simulink library "carnot"  (R2018b)
settings: Solver=VariableStepAuto  StartTime=0.0  StopTime=10.0  RelTol=1e-3
undefined symbols (not defined in the file or in its folder): A, A_earth, acol, Acol, ActPower1, ActPower2, ActPower3, Ad, Ad0, Ar, Au, Au0, Azimuth_Angle, B, Bd, Bd0, Br, Bu, Bu0, C, c1, c2, c3, c33, c4, c5, c6, CarnotCallbacks_Density, CarnotCallbacks_Enthalpy, CarnotCallbacks_Enthalpy2Temperature, CarnotCallbacks_Entropy, CarnotCallbacks_Evaporation_Enthalpy, CarnotCallbacks_GlobalMessageLevel, CarnotCallbacks_Grashof, CarnotCallbacks_Heat_Capacity, CarnotCallbacks_Kinematic_Viscosity, CarnotCallbacks_PMV_PPD, CarnotCallbacks_Prandtl, CarnotCallbacks_Saturation_Property, CarnotCallbacks_Saturation_Temperature, CarnotCallbacks_Saturation_Value_Water, CarnotCallbacks_Specific_Volume, CarnotCallbacks_Thermal_Conductivity, CarnotCallbacks_Vapour_Content, CarnotCallbacks_Vapour_Pressure, Cd, Cdl, Cr, Cu, Davies, Dd, DE_TRY2010_04_averageYear, delta_grd, density, DiameterLastPiece, dl, DPConstant, DPLinear, DPQuadratic, Dr ... (+59)
libraries: $bdroot x429, simulink x36, simulink_extras x12
(part 15 of 22)

== system carnot/Load/Hot_Water_Tapping/mdot_annual_profile ==
  note: Don't change any names
      | in this subsystem!
  Gain : Gain  Gain=1/10000  SaturateOnIntegerOverflow=on  OutDataTypeStr=Inherit: Same as input  ParamDataTypeStr=Inherit: Same as input
  Multiport Switch : MultiPortSwitch  Inputs=2  SaturateOnIntegerOverflow=on  InputSameDT=on
  Product : Product  Inputs=3  SaturateOnIntegerOverflow=on  InputSameDT=on  OutDataTypeStr=Inherit: Same as first input
  RS Month : simulink/Sources/Repeating Sequence  rep_seq_t=[0 2678399 2678399+1 5097599 5097599+1 7775999 7775999+1 10367999 10367999+1 13046399 13046399+1 15638399 15638399+1 18316799 18316799+1 20995199 20995199+1 23587199 23587199+1 26265599 26265599+1 28857599 28857599+1 31536000]  rep_seq_y=[99 99 97 97 100 100 100 100 103 103 105 105 109 109 112 112 108 108 105 105 101 101 100 100]
  RS Sunday : simulink/Sources/Repeating Sequence  rep_seq_t="100*[0 18 18+1 36 36+1 54 54+1 72 72+1 90 90+1 108 108+1 126 126+1 144 144+1 162 162+1 180 180+1 198 198+1 216 216+1 234 234+1 252 252+1 270 270+1 288 288+1 306 306+1 324 324+1 342 342+1 360 360+1 378 378+1 396 396+1 414 414+1 432 432+1 450 450+1 468 468+1 486 486+1 504 504+1 522 522+1 540 540+1 558 558+1 576 576+1 594 594+1 612 612+1 630 630+1 648 648+1 666 666+1 684 684+1 702 702+1 720 720+1 738 738+1 756 756+1 774 774+1 792 792+1 810 810+1 828 828+1 846 846+1  864]"  rep_seq_y=[0 0 0 0 0.5 0.5 0.5 0.5 0.5 0.5 0.5 0.5 1 1 1 1 1 1 1 1 1 1 1 1 1 1 2 2 2 2 3 3 2 2 2 2 2 2 2 2 3 3 2 2 2 2 2 2 3 3 3 3 3 3 3 3 3 3 2 2 2 2 1 1 1 1 2 2 2 2 3 3 3 3 3 3 3 3 2 2 2 2 2 2 2 2 2 2 1 1 1 1 1 1 1 1]
  RS Weekday : simulink/Sources/Repeating Sequence  rep_seq_t="100*[0 18 18+1 36 36+1 54 54+1 72 72+1 90 90+1 108 108+1 126 126+1 144 144+1 162 162+1 180 180+1 198 198+1 216 216+1 234 234+1 252 252+1 270 270+1 288 288+1 306 306+1 324 324+1 342 342+1 360 360+1 378 378+1 396 396+1 414 414+1 432 432+1 450 450+1 468 468+1 486 486+1 504 504+1 522 522+1 540 540+1 558 558+1 576 576+1 594 594+1 612 612+1 630 630+1 648 648+1 666 666+1 684 684+1 702 702+1 720 720+1 738 738+1 756 756+1 774 774+1 792 792+1 810 810+1 828 828+1 846 846+1  864]"  rep_seq_y=[0.5 0.5 0.5 0.5 0.5 0.5 0.5 0.5 0.5 0.5 0.5 0.5 1 1 1 1 1 1 1 1 2 2 2 2 3 3 3 3 5 5 5 5 5 5 5 5 4 4 4 4 3 3 2 2 2 2 2 2 3 3 3 3 4 4 4 4 3 3 2 2 2 2 1 1 1 1 2 2 2 2 3 3 3 3 3 3 3 3 2 2 2 2 2 2 2 2 2 2 1 1 1 1 1 1 1 1]
  Repeating Sequence Day of the Week : simulink/Sources/Repeating Sequence  rep_seq_t=[0 5*24*3600 5*24*3600+1 7*24*3600]  rep_seq_y=[1 1 2 2]
  mdot0 : Constant  Value=0.1
  mdot : Outport
  wires:
  RS Month/1 -> Product/2
  RS Weekday/1 -> Multiport Switch/2
  Gain/1 -> mdot/1
  Product/1 -> Gain/1
  mdot0/1 -> Product/1
  Multiport Switch/1 -> Product/3
  RS Sunday/1 -> Multiport Switch/3
  Repeating Sequence Day of the Week/1 -> Multiport Switch/1

== system carnot/Load/Hot_Water_Tapping/mdot_rep_seq ==
  Add : Sum  Inputs=1
  Pulse Generator : DiscretePulseGenerator  PulseType=Time based  Amplitude=rep_seq_y  Period=period  PulseWidth=rep_seq_d*100/period  PhaseDelay=rep_seq_t
  Out1 : Outport
  wires:
  Pulse Generator/1 -> Add/1
  Add/1 -> Out1/1

== system carnot/Load/Houses/House_simple ==
  WDB : Inport
  THB : Inport  Port=2
  RDB : Inport  Port=3
  Ahabit : Constant  Value=Ahabit
  AirComposition : Subsystem
  Bus Creator : BusCreator  Inputs=8
  Bus Selector1 : BusSelector  OutputSignals=Sunshade,OpenWindow,Qdot_internal
  Bus Selector2 : BusSelector  OutputSignals=CalculateAirComposition
  Constant1 : Constant  Value=20
  HeatTransfer2Ground_ISO13370 : $bdroot/Basic/Heat_Transfer/HeatTransfer2Ground_ISO13370  slabwidth=slabwidth  slablength=slablength  gammat=gammat  Tmeaninside=Tmeaninside  deltathetai=deltathetai  Tmeanoutside=Tmeanoutside  deltathetae=deltathetae  tshift=tshift  dwall=dwall  cond_ground=cond_ground  cp_ground=cp_ground  rho_ground=rho_ground  utot=utot
  House_OneNodeModel : $bdroot/Basic/Thermal_Models/House_OneNodeModel  A=Ahabit  UAout=UAwall  UAin=0  capa=capa  tini=tini  dtroom=dtroom  AziWin=AziWin  Awin=Awindow  Uwin=Uwindow  Gwin=Gwindow
  Radiator : $bdroot/Source/Heat_Exchanger/Radiator  pnom=pnom  dtnom=dtnom  expo=expo  mcap=mcap  tini=tini  lin=lin  qua=qua
  Ventilation : $bdroot/Source/Ventilation/Ventilation  Ahabit=Ahabit  Hroom=Hroom  vent=Ventilationrate  rec=Heatrecovery  ppmCO2=400  ppmVOC=0  alpha=alpha  H=H  W=W  Nwin=Nwin
  Hdat : Outport
  THBout : Outport  Port=2
  wires:
  Ventilation/2 -> AirComposition/1(THBvent)
  AirComposition/1(AirComp) -> Bus Creator/8  "AirComposition"
  Bus Selector2/1 -> AirComposition/Enable  "<CalculateAirComposition>"
  Ahabit/1 -> Bus Creator/7  "Ahabit"
  THB/1 -> Radiator/2, Bus Creator/5  "THB_in"
  Radiator/2 -> THBout/1, Bus Creator/6  "THB_out"
  House_OneNodeModel/1 -> Ventilation/2, Radiator/1, Bus Creator/1  "Troom"
  House_OneNodeModel/2 -> Bus Creator/2  "Qdot"
  Bus Creator/1 -> Hdat/1
  HeatTransfer2Ground_ISO13370/1 -> House_OneNodeModel/5
  Constant1/1 -> House_OneNodeModel/1
  Bus Selector1/3 -> House_OneNodeModel/6  "<Qdot_internal>"
  Radiator/1 -> House_OneNodeModel/7  "Qdot"
  Ventilation/1 -> House_OneNodeModel/4
  WDB/1 -> Ventilation/1, House_OneNodeModel/2, Bus Creator/4  "WDB"
  RDB/1 -> Bus Selector1/1, Bus Selector2/1, AirComposition/2(RDB), Bus Creator/3  "RDB"
  Bus Selector1/1 -> House_OneNodeModel/3  "<Sunshade>"
  Bus Selector1/2 -> Ventilation/3  "<OpenWindow>"

== system carnot/Load/Houses/Resident_Data ==
  Qdot_internal : Inport
  Sunshade : Inport  Port=2
  OpenWindow : Inport  Port=3
  Massflow_CO2 : Inport  Port=4
  Massflow_H2O : Inport  Port=5
  Massflow_VOC : Inport  Port=6
  Bus Creator : BusCreator  Inputs=7
  CalculateAirComposition : Constant  Value=CalcAirComp  mask{CalcAirComp=on}
      mask prompts: CalcAirComp "Calculate the composition of room air (H2O, CO2, VOC)"
  RDB : Outport
  wires:
  CalculateAirComposition/1 -> Bus Creator/4  "CalculateAirComposition"
  Massflow_VOC/1 -> Bus Creator/7  "Massflow_VOC"
  Massflow_H2O/1 -> Bus Creator/6  "Massflow_H2O"
  Massflow_CO2/1 -> Bus Creator/5  "Massflow_CO2"
  Qdot_internal/1 -> Bus Creator/1  "Qdot_internal"
  OpenWindow/1 -> Bus Creator/3  "OpenWindow"
  Bus Creator/1 -> RDB/1
  Sunshade/1 -> Bus Creator/2  "Sunshade"

== system carnot/Load/Houses/Resident_Task44 ==
  WDB : Inport
  Troom : Inport  Port=2
  Bus Creator : BusCreator  Inputs=7
  Bus Selector : BusSelector  OutputSignals=Temperature_Ambient
  CalculateAirComposition : Constant  Value=CalcAirComp  mask{CalcAirComp=off}
      mask prompts: CalcAirComp "Calculate the composition of room air (H2O, CO2, VOC)"
  Electric_Gains_Profile : $bdroot/Load/General/Repeating_Profile  period=period  rep_seq_t=rep_seq_te  rep_seq_d=rep_seq_de  rep_seq_y=rep_seq_ye
  Massflow_CO2 : Constant  Value=mdotCO2
  Massflow_H2O : Constant  Value=mdotH2O
  Massflow_VOC : Constant  Value=mdotVOC
  Occupation_Profile : $bdroot/Load/General/Repeating_Profile  period=period  rep_seq_t=rep_seq_to  rep_seq_d=rep_seq_do  rep_seq_y=rep_seq_yo
  Shading_Control : $bdroot/Control/Shading_Control  TroomShadeOn=TroomShadeOn  TroomShadeOff=TroomShadeOff  SolarShadeOn=SolarShadeOn  SolarShadeOff=SolarShadeOff  max_shade=max_shade
  Window_Control : $bdroot/Control/Window_Control  Topen=Topen  Tclose=Tclose  TrAboveTa=TrAboveTa  TaTooCold=TaTooCold  timeFIR=timeFIR  TaIni=TaIni  starttime=starttime  stoptime=stoptime
  add : Sum  Inputs=2
  RDB : Outport
  wires:
  CalculateAirComposition/1 -> Bus Creator/4  "CalculateAirComposition"
  Massflow_VOC/1 -> Bus Creator/7  "Massflow_VOC"
  Massflow_H2O/1 -> Bus Creator/6  "Massflow_H2O"
  Massflow_CO2/1 -> Bus Creator/5  "Massflow_CO2"
  Occupation_Profile/1 -> add/1
  Electric_Gains_Profile/1 -> add/2
  add/1 -> Bus Creator/1  "Qdot_internal"
  Window_Control/1 -> Bus Creator/3  "OpenWindow"
  Bus Creator/1 -> RDB/1
  Shading_Control/1 -> Bus Creator/2  "Sunshade"
  Bus Selector/1 -> Window_Control/1  "<Temperature_Ambient>"
  Troom/1 -> Window_Control/2, Shading_Control/2
  WDB/1 -> Bus Selector/1, Shading_Control/1

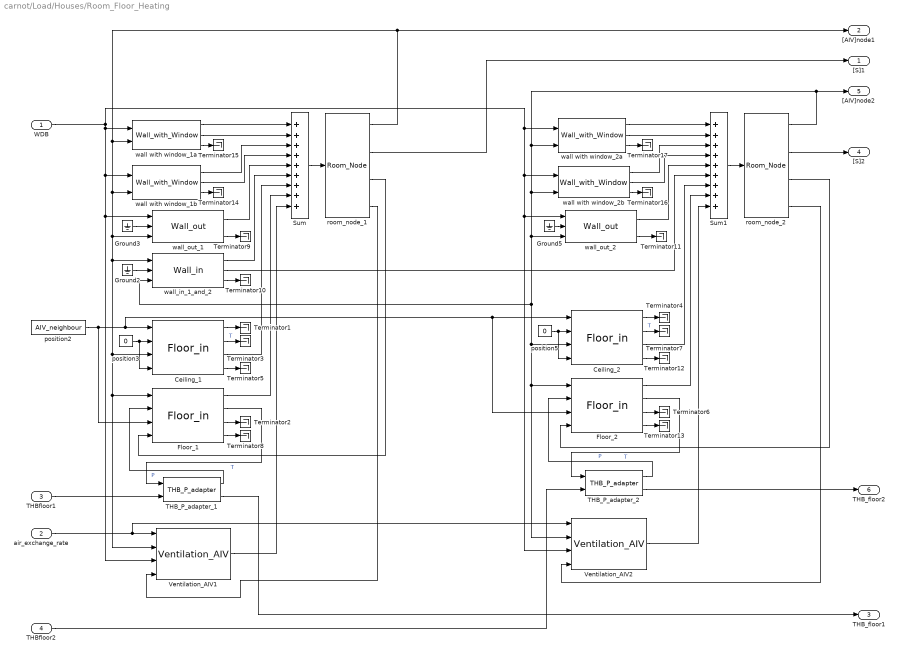
== system carnot/Load/Houses/Room_Floor_Heating ==
  WDB : Inport
  air_exchange_rate : Inport  Port=2
  THBfloor1 : Inport  Port=3
  THBfloor2 : Inport  Port=4
  Ceiling_1 : $bdroot/Basic/Thermal_Models/Floor_in  wallsize=[5 5]  t0=20  d=[0.015 0.38 0.02]  cond=[1.4 0.79 0.7]  cwall=[0.28 0.28 0.28]*3600  rho=[2000 1800 1400]  misc=[0.9 0.9]  dactive=-1  tau=1000*3600
  Ceiling_2 : $bdroot/Basic/Thermal_Models/Floor_in  wallsize=[5 5]  t0=20  d=[0.015 0.38 0.02]  cond=[1.4 0.79 0.7]  cwall=[0.28 0.28 0.28]*3600  rho=[2000 1800 1400]  misc=[0.9 0.9]  dactive=-1  tau=1000*3600
  Floor_1 : $bdroot/Basic/Thermal_Models/Floor_in  wallsize=[5 5]  t0=20  d=[0.015 0.38 0.02]  cond=[1.4 0.79 0.7]  cwall=[0.28 0.28 0.28]*3600  rho=[2000 1800 1400]  misc=[0.9 0.9]  dactive=0.02  tau=1000*3600
  Floor_2 : $bdroot/Basic/Thermal_Models/Floor_in  wallsize=[5 5]  t0=20  d=[0.015 0.38 0.02]  cond=[1.4 0.79 0.7]  cwall=[0.28 0.28 0.28]*3600  rho=[2000 1800 1400]  misc=[0.9 0.9]  dactive=0.02  tau=1000*3600
  Ground2 : Ground
  Ground3 : Ground
  Ground5 : Ground
  Sum : Sum  Inputs=9  SaturateOnIntegerOverflow=on  InputSameDT=on  OutDataTypeStr=Inherit: Same as first input
  Sum1 : Sum  Inputs=9  SaturateOnIntegerOverflow=on  InputSameDT=on  OutDataTypeStr=Inherit: Same as first input
  THB_P_adapter_1 : $bdroot/Source/Heat_Exchanger/THB_P_adapter  mass=1  ua=800*5*5/0.2*0.022*3.1415  t0=20
  THB_P_adapter_2 : $bdroot/Source/Heat_Exchanger/THB_P_adapter  mass=1  ua=800*5*5/0.2*0.022*3.1415  t0=20
  Terminator{1..17} (17 alike) : Terminator
  Ventilation_AIV1 : $bdroot/Source/Ventilation/Ventilation_AIV  co2=400
  Ventilation_AIV2 : $bdroot/Source/Ventilation/Ventilation_AIV  co2=400
  position2 : Constant  Value=AIV_neighbour
  position3 : Constant  Value=0
  position5 : Constant  Value=0
  room_node_1 : $bdroot/Basic/Thermal_Models/Room_Node  zoneairvolume=5*5*2.5  zoneheight=2.5  zonestartTEMP=20  zonestartWATER=55  timeconst=100  heatperfect=natural  lookuptime=[0 24]*3600  lookupvalue=[20 20]  AirPressure=101300  calc_p=off
  room_node_2 : $bdroot/Basic/Thermal_Models/Room_Node  zoneairvolume=5*5*2.5  zoneheight=2.5  zonestartTEMP=20  zonestartWATER=55  timeconst=100  heatperfect=natural  lookuptime=[0 24]*3600  lookupvalue=[20 20]  AirPressure=101300  calc_p=off
  wall with window_1a : $bdroot/Basic/Thermal_Models/Wall_with_Window  wallsize=[2.5 5]  windowsize=[1 2]  frame=0.1  pos=90  t0=20  tau=1000*3600  g=0.7
  wall with window_1b : $bdroot/Basic/Thermal_Models/Wall_with_Window  wallsize=[2.5 5]  windowsize=[1 2]  frame=0.1  pos=0  t0=20  tau=1000*3600  g=0.7
  wall with window_2a : $bdroot/Basic/Thermal_Models/Wall_with_Window  wallsize=[2.5 5]  windowsize=[1 2]  frame=0.1  pos=-90  t0=20  tau=1000*3600  g=0.7
  wall with window_2b : $bdroot/Basic/Thermal_Models/Wall_with_Window  wallsize=[2.5 5]  windowsize=[1 2]  frame=0.1  pos=0  t0=20  tau=1000*3600  g=0.7
  wall_in_1_and_2 : $bdroot/Basic/Thermal_Models/Wall_in  wallsize=[2.5 5]  d=[0.015 0.38 0.02]  cond=[1.4 0.79 0.7]  cwall=[0.28 0.28 0.28]*3600  rho=[2000 1800 1400]  emission_in=.96  dactive=-1  t0=20  tau=1000*3600
  wall_out_1 : $bdroot/Basic/Thermal_Models/Wall_out  wallsize=[2.5 5]  pos=180  t0=20  d=[0.1 0.38]  cond=[0.04 0.79]  cwall=[0.28 0.28]*3600  rho=[900 1800]  reflectground=0.2  abs_emiss=[0.65 0.97 0.96]  tau=1000*3600  dactive=-1
  wall_out_2 : $bdroot/Basic/Thermal_Models/Wall_out  wallsize=[2.5 5]  pos=180  t0=20  d=[0.1 0.38]  cond=[0.04 0.79]  cwall=[0.28 0.28]*3600  rho=[900 1800]  reflectground=0.2  abs_emiss=[0.65 0.97 0.96]  tau=1000*3600  dactive=-1
  "[S]1" : Outport
  "[AIV]node1" : Outport  Port=2
  THB_floor1 : Outport  Port=3
  "[S]2" : Outport  Port=4
  "[AIV]node2" : Outport  Port=5
  THB_floor2 : Outport  Port=6
  wires:
  Sum1/1 -> room_node_2/1
  Sum/1 -> room_node_1/1
  room_node_2/1 -> "[AIV]node2"/1, wall with window_2a/2, wall_in_1_and_2/3, Ceiling_2/3, Ventilation_AIV2/2, Floor_2/1, wall_out_2/3, wall with window_2b/2
  room_node_1/1 -> "[AIV]node1"/1, wall_out_1/3, Ventilation_AIV1/2, Floor_1/1, Ceiling_1/3, wall_in_1_and_2/1, wall with window_1b/2, wall with window_1a/2
  air_exchange_rate/1 -> Ventilation_AIV1/1, Ventilation_AIV2/1
  wall_in_1_and_2/2 -> Sum1/6
  Ground5/1 -> wall_out_2/2
  room_node_2/3 -> Floor_2/4
  room_node_2/4 -> Ventilation_AIV2/4
  THB_P_adapter_2/2 -> THB_floor2/1
  THB_P_adapter_2/1 -> Floor_2/2  "P"
  Floor_2/2 -> THB_P_adapter_2/1  "T"
  THBfloor2/1 -> THB_P_adapter_2/2
  Ventilation_AIV2/1 -> Sum1/9
  Ceiling_2/3 -> Sum1/7
  Floor_2/1 -> Sum1/8
  position5/1 -> Ceiling_2/2, Ceiling_2/4
  Floor_2/3 -> Terminator6/1
  Ceiling_2/2 -> Terminator7/1  "T"
  Ceiling_2/1 -> Terminator4/1
  room_node_2/2 -> "[S]2"/1
  wall with window_2b/2 -> Sum1/4
  wall_out_2/1 -> Sum1/5
  wall with window_2b/1 -> Sum1/3
  wall with window_2a/2 -> Sum1/2
  wall with window_2a/1 -> Sum1/1
  position2/1 -> Ceiling_2/1, Floor_2/3, Ceiling_1/1, Floor_1/3
  Ground3/1 -> wall_out_1/2
  Ground2/1 -> wall_in_1_and_2/2
  room_node_1/3 -> Floor_1/4
  room_node_1/4 -> Ventilation_AIV1/4
  THB_P_adapter_1/2 -> THB_floor1/1
  THB_P_adapter_1/1 -> Floor_1/2  "P"
  Floor_1/2 -> THB_P_adapter_1/1  "T"
  THBfloor1/1 -> THB_P_adapter_1/2
  Ventilation_AIV1/1 -> Sum/9
  Ceiling_1/3 -> Sum/7
  Floor_1/1 -> Sum/8
  position3/1 -> Ceiling_1/4, Ceiling_1/2
  Floor_1/3 -> Terminator2/1
  Ceiling_1/2 -> Terminator3/1  "T"
  Ceiling_1/1 -> Terminator1/1
  room_node_1/2 -> "[S]1"/1
  wall with window_1b/2 -> Sum/4
  wall_out_1/1 -> Sum/5
  wall with window_1b/1 -> Sum/3
  wall with window_1a/2 -> Sum/2
  wall with window_1a/1 -> Sum/1
  WDB/1 -> wall with window_1a/1, Ventilation_AIV1/3, wall_out_1/1, wall with window_1b/1, Ventilation_AIV2/3, wall_out_2/1, wall with window_2b/1, wall with window_2a/1
  wall_in_1_and_2/1 -> Sum/6
  Ceiling_1/4 -> Terminator5/1
  Floor_1/4 -> Terminator8/1
  wall_out_1/2 -> Terminator9/1
  wall_in_1_and_2/3 -> Terminator10/1
  wall_out_2/2 -> Terminator11/1
  Ceiling_2/4 -> Terminator12/1
  Floor_2/4 -> Terminator13/1
  wall with window_1b/3 -> Terminator14/1
  wall with window_1a/3 -> Terminator15/1
  wall with window_2b/3 -> Terminator16/1
  wall with window_2a/3 -> Terminator17/1

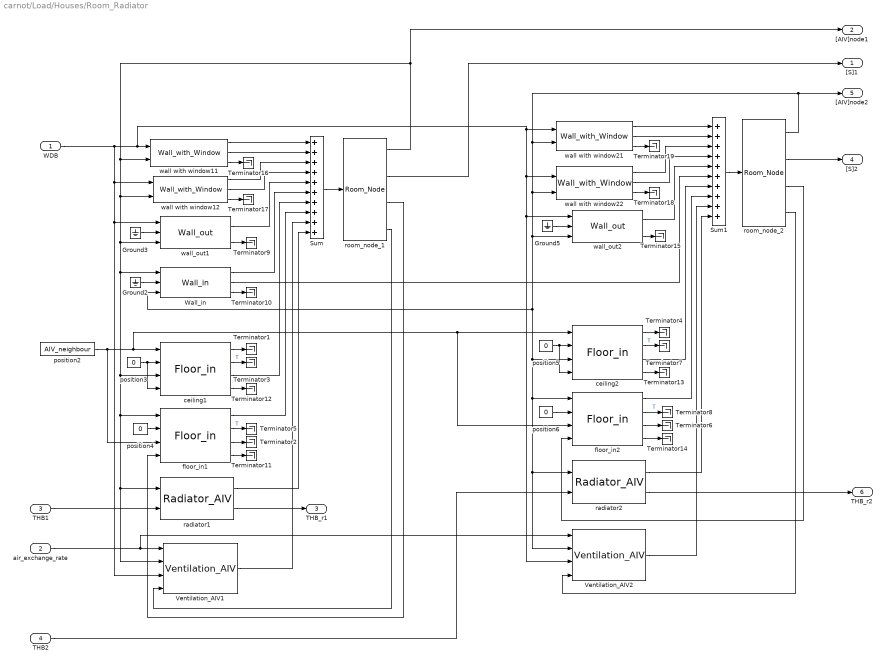
== system carnot/Load/Houses/Room_Radiator ==
  WDB : Inport
  air_exchange_rate : Inport  Port=2
  THB1 : Inport  Port=3
  THB2 : Inport  Port=4
  Ground2 : Ground
  Ground3 : Ground
  Ground5 : Ground
  Sum : Sum  Inputs=10  SaturateOnIntegerOverflow=on  InputSameDT=on  OutDataTypeStr=Inherit: Same as first input
  Sum1 : Sum  Inputs=10  SaturateOnIntegerOverflow=on  InputSameDT=on  OutDataTypeStr=Inherit: Same as first input
  Terminator{1..19} (19 alike) : Terminator
  Ventilation_AIV1 : $bdroot/Source/Ventilation/Ventilation_AIV  co2=400
  Ventilation_AIV2 : $bdroot/Source/Ventilation/Ventilation_AIV  co2=400
  Wall_in : $bdroot/Basic/Thermal_Models/Wall_in  wallsize=[2.5 5]  d=[0.015 0.38 0.02]  cond=[1.4 0.79 0.7]  cwall=[0.28 0.28 0.28]*3600  rho=[2000 1800 1400]  emission_in=0.96  dactive=-1  t0=20  tau=1000*3600
  ceiling1 : $bdroot/Basic/Thermal_Models/Floor_in  wallsize=[5 5]  t0=20  d=[0.015 0.38 0.02]  cond=[1.4 0.79 0.7]  cwall=[0.28 0.28 0.28]*3600  rho=[2000 1800 1400]  misc=[0.9 0.9]  dactive=-1  tau=1000*3600
  ceiling2 : $bdroot/Basic/Thermal_Models/Floor_in  wallsize=[5 5]  t0=20  d=[0.015 0.38 0.02]  cond=[1.4 0.79 0.7]  cwall=[0.28 0.28 0.28]*3600  rho=[2000 1800 1400]  misc=[0.9 0.9]  dactive=-1  tau=1000*3600
  floor_in1 : $bdroot/Basic/Thermal_Models/Floor_in  wallsize=[5 5]  t0=20  d=[0.015 0.38 0.02]  cond=[1.4 0.79 0.7]  cwall=[0.28 0.28 0.28]*3600  rho=[2000 1800 1400]  misc=[0.9 0.9]  dactive=-1  tau=1000*3600
  floor_in2 : $bdroot/Basic/Thermal_Models/Floor_in  wallsize=[5 5]  t0=20  d=[0.015 0.38 0.02]  cond=[1.4 0.79 0.7]  cwall=[0.28 0.28 0.28]*3600  rho=[2000 1800 1400]  misc=[0.9 0.9]  dactive=-1  tau=1000*3600
  position2 : Constant  Value=AIV_neighbour
  position{3..6} (4 alike) : Constant  Value=0
  radiator1 : $bdroot/Source/Heat_Exchanger/Radiator_AIV  pnom=500  dtnom=40  expo=1.3  mcap=5*4182  ra=0.47  tini=20  lin=0  qua=1000
  radiator2 : $bdroot/Source/Heat_Exchanger/Radiator_AIV  pnom=500  dtnom=40  expo=1.3  mcap=5*4182  ra=0.47  tini=20  lin=0  qua=1000
  room_node_1 : $bdroot/Basic/Thermal_Models/Room_Node  zoneairvolume=5*5*2.5  zoneheight=2.5  zonestartTEMP=20  zonestartWATER=55  timeconst=100  heatperfect=natural  lookuptime=[0 24]*3600  lookupvalue=[20 20]  AirPressure=101300  calc_p=off
  room_node_2 : $bdroot/Basic/Thermal_Models/Room_Node  zoneairvolume=5*5*2.5  zoneheight=2.5  zonestartTEMP=20  zonestartWATER=55  timeconst=100  heatperfect=natural  lookuptime=[0 24]*3600  lookupvalue=[20 20]  AirPressure=101300  calc_p=off
  wall with window11 : $bdroot/Basic/Thermal_Models/Wall_with_Window  wallsize=[2.5 5]  windowsize=[1 2]  frame=0.1  pos=90  t0=20  tau=1000*3600  g=0.7
  wall with window12 : $bdroot/Basic/Thermal_Models/Wall_with_Window  wallsize=[2.5 5]  windowsize=[1 2]  frame=0.1  pos=0  t0=20  tau=1000*3600  g=0.7
  wall with window21 : $bdroot/Basic/Thermal_Models/Wall_with_Window  wallsize=[2.5 5]  windowsize=[1 2]  frame=0.1  pos=-90  t0=20  tau=1000*3600  g=0.7
  wall with window22 : $bdroot/Basic/Thermal_Models/Wall_with_Window  wallsize=[2.5 5]  windowsize=[1 2]  frame=0.1  pos=0  t0=20  tau=1000*3600  g=0.7
  wall_out1 : $bdroot/Basic/Thermal_Models/Wall_out  wallsize=[2.5 5]  pos=180  t0=20  d=[0.1 0.38]  cond=[0.04 0.79]  cwall=[0.28 0.28]*3600  rho=[900 1800]  reflectground=0.2  abs_emiss=[0.65 0.97 0.96]  tau=1000*3600  dactive=-1
  wall_out2 : $bdroot/Basic/Thermal_Models/Wall_out  wallsize=[2.5 5]  pos=180  t0=20  d=[0.1 0.38]  cond=[0.04 0.79]  cwall=[0.28 0.28]*3600  rho=[900 1800]  reflectground=0.2  abs_emiss=[0.65 0.97 0.96]  tau=1000*3600  dactive=-1
  "[S]1" : Outport
  "[AIV]node1" : Outport  Port=2
  THB_r1 : Outport  Port=3
  "[S]2" : Outport  Port=4
  "[AIV]node2" : Outport  Port=5
  THB_r2 : Outport  Port=6
  wires:
  Sum1/1 -> room_node_2/1
  Sum/1 -> room_node_1/1
  radiator2/1 -> Sum1/10
  radiator1/1 -> Sum/10
  position6/1 -> floor_in2/2
  position4/1 -> floor_in1/2
  floor_in1/2 -> Terminator5/1  "T"
  floor_in2/2 -> Terminator8/1  "T"
  room_node_2/1 -> "[AIV]node2"/1, wall with window21/2, wall with window22/2, ceiling2/3, Ventilation_AIV2/2, radiator2/1, floor_in2/1, Wall_in/3, wall_out2/3
  room_node_1/1 -> "[AIV]node1"/1, Ventilation_AIV1/2, radiator1/1, floor_in1/1, ceiling1/3, Wall_in/1, wall_out1/3, wall with window12/2, wall with window11/2
  air_exchange_rate/1 -> Ventilation_AIV2/1, Ventilation_AIV1/1
  Wall_in/2 -> Sum1/6
  Ground5/1 -> wall_out2/2
  room_node_2/3 -> floor_in2/4
  room_node_2/4 -> Ventilation_AIV2/4
  radiator2/2 -> THB_r2/1
  THB2/1 -> radiator2/2
  Ventilation_AIV2/1 -> Sum1/9
  ceiling2/3 -> Sum1/7
  floor_in2/1 -> Sum1/8
  position5/1 -> ceiling2/2, ceiling2/4
  floor_in2/3 -> Terminator6/1
  ceiling2/2 -> Terminator7/1  "T"
  ceiling2/1 -> Terminator4/1
  room_node_2/2 -> "[S]2"/1
  wall with window22/2 -> Sum1/4
  wall_out2/1 -> Sum1/5
  wall with window22/1 -> Sum1/3
  wall with window21/2 -> Sum1/2
  wall with window21/1 -> Sum1/1
  position2/1 -> ceiling2/1, floor_in2/3, ceiling1/1, floor_in1/3
  Ground3/1 -> wall_out1/2
  Ground2/1 -> Wall_in/2
  room_node_1/3 -> floor_in1/4
  room_node_1/4 -> Ventilation_AIV1/4
  radiator1/2 -> THB_r1/1
  THB1/1 -> radiator1/2
  Ventilation_AIV1/1 -> Sum/9
  ceiling1/3 -> Sum/7
  floor_in1/1 -> Sum/8
  position3/1 -> ceiling1/4, ceiling1/2
  floor_in1/3 -> Terminator2/1
  ceiling1/2 -> Terminator3/1  "T"
  ceiling1/1 -> Terminator1/1
  room_node_1/2 -> "[S]1"/1
  wall with window12/2 -> Sum/4
  wall_out1/1 -> Sum/5
  wall with window12/1 -> Sum/3
  wall with window11/2 -> Sum/2
  wall with window11/1 -> Sum/1
  WDB/1 -> Ventilation_AIV2/3, wall_out2/1, wall with window22/1, wall with window21/1, wall with window11/1, Ventilation_AIV1/3, wall_out1/1, wall with window12/1
  Wall_in/1 -> Sum/6
  wall_out1/2 -> Terminator9/1
  Wall_in/3 -> Terminator10/1
  floor_in1/4 -> Terminator11/1
  ceiling1/4 -> Terminator12/1
  ceiling2/4 -> Terminator13/1
  floor_in2/4 -> Terminator14/1
  wall_out2/2 -> Terminator15/1
  wall with window11/3 -> Terminator16/1
  wall with window12/3 -> Terminator17/1
  wall with window22/3 -> Terminator18/1
  wall with window21/3 -> Terminator19/1

== system carnot/Source/Boiler/Condensing_Boiler ==
  Tamb : Inport
  THBin : Inport  Port=2
  Ctrl : Inport  Port=3
  Fuel : Inport  Port=4
  Bus Assignment : BusAssignment  AssignedSignals=Temperature
  Bus Creator : BusCreator  Inputs=7
  Bus Selector : BusSelector  OutputSignals=Temperature,MassFlow,Pressure
  Bus Selector1 : BusSelector  OutputSignals=FluidType,FluidMix  OutputAsBus=on
  Bus Selector2 : BusSelector  OutputSignals=Fuel_ID
  Bus Selector3 : BusSelector  OutputSignals=Temperature
  Combustion_Calculation : $bdroot/Basic/Thermal_Models/Combustion_Calculation  SystemSampleTime=-1
  Pgas : Gain  Gain=Pgas
  PowerMeter : $bdroot/Control/PowerMeter
  Pressure_Drop_Fix : $bdroot/Basic/Pressure_Drop/Pressure_Drop_Fix  con=0  lin=dplin  qua=dpqua
  Product : Product  RndMeth=Zero
  SelectTefficiency : Subsystem  mask{whichTforEfficiency=mean of inlet and outlet temperature}
      mask prompts: whichTforEfficiency "Efficiency based on :"
      mask TypeOptions whichTforEfficiency: mean of inlet and outlet temperature | inlet temperature | outlet temperature
  TableEfficiency : Lookup_n-D  BreakpointsForDimension1=TableRelativePower  BreakpointsForDimension2=TableTemperatures  Table=TableData  InternalRulePriority=Speed  RndMeth=Simplest  InputSameDT=on
  TablePelec : Lookup_n-D  NumberOfTableDimensions=1  BreakpointsForDimension1=TableRelativePower  Table=ElectricPower  InternalRulePriority=Speed  RndMeth=Simplest  InputSameDT=on
  limitCtrl : Subsystem  mask{relQdotMin=relQdotMin}
      mask prompts: relQdotMin "Minimum control signal for "ON""
  sfunBoiler : $bdroot/Basic/Thermal_Models/sfunBoiler  UA=HeatLoss  vol=Volume  Tini=Tini  nodes=nodes
  THB : Outport
  Bdat : Outport  Port=2
  wires:
  Bus Selector3/1 -> SelectTefficiency/2(Tin)  "<Temperature>"
  SelectTefficiency/2(Teff) -> TableEfficiency/2
  SelectTefficiency/1(Tmean) -> Bus Creator/3, Combustion_Calculation/4  "Tmean"
  Combustion_Calculation/1 -> Bus Creator/5  "eco"
  PowerMeter/1 -> Bus Creator/4  "Qdot"
  TablePelec/1 -> Combustion_Calculation/3
  Bus Creator/1 -> Bdat/1  "Bdat"
  Bus Selector1/1 -> sfunBoiler/5  "[fluid_type fluid_mix]"
  THBin/1 -> Bus Creator/1, PowerMeter/2, Pressure_Drop_Fix/1, Bus Selector/1, Bus Selector1/1, Bus Selector3/1  "THBin"
  Bus Selector/2 -> sfunBoiler/3  "<MassFlow>"
  Bus Assignment/1 -> Bus Creator/2, PowerMeter/1, THB/1  "THBout"
  Bus Selector/3 -> sfunBoiler/4  "<Pressure>"
  Tamb/1 -> sfunBoiler/1
  Bus Selector/1 -> sfunBoiler/2  "<Temperature>"
  sfunBoiler/1 -> Bus Assignment/2, SelectTefficiency/1(Tout)  "Tout"
  Fuel/1 -> Bus Selector2/1, Combustion_Calculation/5
  TableEfficiency/1 -> Combustion_Calculation/2, Product/1
  limitCtrl/1(Out1) -> Pgas/1, TableEfficiency/1, TablePelec/1, Bus Creator/6  "ControlActual"
  Product/1 -> sfunBoiler/6
  Bus Selector2/1 -> Combustion_Calculation/Enable  "<Fuel_ID>"
  Pressure_Drop_Fix/1 -> Bus Assignment/1
  Pgas/1 -> Combustion_Calculation/1, Product/2
  Ctrl/1 -> limitCtrl/1(In1), Bus Creator/7  "ControlSetpoint"

== system carnot/Source/Boiler/Electric_Heater ==
  THBin : Inport
  Heating_Power : Inport  Port=2
  Bus Assignment : BusAssignment  AssignedSignals=Temperature
  Bus Selector : BusSelector  OutputSignals=MassFlow
  Bus Selector1 : BusSelector  OutputSignals=Temperature
  Heat_Capacity : $bdroot/Basic/Material_Properties/Heat_Capacity  VariantControl=CarlibClassic  INPUTARGUMENTS=THB  DEBUGLEVEL=DEBUGLEVEL  MAXTOTALWARNINGS=inf  MAXCONSECUTIVEWARNINGS=inf  WRITETOFILE=0  FILENAME='errors.txt'
  Product : Product  Inputs=//*  SaturateOnIntegerOverflow=on  InputSameDT=on  OutDataTypeStr=Inherit: Same as first input
  Saturation : Saturate  UpperLimit=inf  LowerLimit=1e-5
  Sum : Sum  SaturateOnIntegerOverflow=on  InputSameDT=on  OutDataTypeStr=Inherit: Same as first input
  Transfer Fcn : TransferFcn  Denominator=[60 1]
  THBout : Outport  InitialOutput=0
  wires:
  Sum/1 -> Bus Assignment/2
  Bus Selector1/1 -> Sum/1  "<Temperature>"
  Bus Selector/1 -> Saturation/1  "<MassFlow>"
  Bus Assignment/1 -> THBout/1
  Transfer Fcn/1 -> Sum/2
  Heating_Power/1 -> Product/3
  Heat_Capacity/1 -> Product/2
  Saturation/1 -> Product/1  "mdot"
  Product/1 -> Transfer Fcn/1
  THBin/1 -> Bus Selector1/1, Bus Selector/1, Heat_Capacity/1, Bus Assignment/1

== system carnot/Source/Boiler/Electric_Heater_Ctrl ==
  THBin : Inport
  Tamb : Inport  Port=2
  Ctrl : Inport  Port=3
  Bus Assignment : BusAssignment  AssignedSignals=Temperature
  Bus Creator : BusCreator  Inputs=5
  Bus Selector : BusSelector  OutputSignals=MassFlow
  Bus Selector1 : BusSelector  OutputSignals=Temperature
  Gain : Gain  Gain=power
  Heat_Capacity : $bdroot/Basic/Material_Properties/Heat_Capacity  VariantControl=CarlibClassic  INPUTARGUMENTS=THB  DEBUGLEVEL=DEBUGLEVEL  MAXTOTALWARNINGS=inf  MAXCONSECUTIVEWARNINGS=inf  WRITETOFILE=0  FILENAME='errors.txt'
  Signal Copy : SignalConversion  OverrideOpt=off
  Thermal_Node : $bdroot/Basic/Thermal_Models/Thermal_Node  UA=UA  mcp=mcp
  THBout : Outport  InitialOutput=0
  EHdat : Outport  Port=2  InitialOutput=0
  wires:
  THBin/1 -> Heat_Capacity/1, Bus Selector/1, Bus Selector1/1, Bus Creator/1, Bus Assignment/1  "THBin"
  Ctrl/1 -> Bus Creator/4, Signal Copy/1, Gain/1  "ControlSetpoint"
  Bus Assignment/1 -> Bus Creator/2, THBout/1  "THBout"
  Bus Selector/1 -> Thermal_Node/3  "<MassFlow>"
  Bus Selector1/1 -> Thermal_Node/2  "<Temperature>"
  Bus Creator/1 -> EHdat/1  "EHdat"
  Gain/1 -> Thermal_Node/4, Bus Creator/3  "Power"
  Signal Copy/1 -> Bus Creator/5  "ControlActual"
  Tamb/1 -> Thermal_Node/1  "Tamb"
  Thermal_Node/1 -> Bus Assignment/2
  Heat_Capacity/1 -> Thermal_Node/5

== system carnot/Source/Chiller/Absorption_Chiller_LookUp ==
  THB_GEN_IN : Inport  OutDataTypeStr=Bus: THB
  THB_COLD_IN : Inport  Port=2  OutDataTypeStr=Bus: THB
  THB_RC_IN : Inport  Port=3  OutDataTypeStr=Bus: THB
  Ctrl : Inport  Port=4
  Bus Creator : BusCreator  Inputs=5
  Bus Selector : BusSelector  OutputSignals=Temperature
  Bus Selector1 : BusSelector  OutputSignals=Temperature
  Bus Selector2 : BusSelector  OutputSignals=Temperature
  Bus Selector3 : BusSelector  OutputSignals=MassFlow
  CompareToZero : simulink/Logic and Bit Operations/Compare To Zero  relop=>  OutDataTypeStr=uint8
  Gain : Gain
  Lookup_table Q_hot + Q_cold + Recooling : Subsystem  TreatAsAtomicUnit=on
  cooling : Subsystem
  el. consumption solutionpump [W] : Gain  Gain=45
  generator : Subsystem
  recooling : Subsystem
  THB_GEN_OUT : Outport
  THB_COLD_OUT : Outport  Port=2
  THB_RC_OUT : Outport  Port=3
  ACdat : Outport  Port=4
  wires:
  Gain/1 -> Bus Creator/5  "ControlActual"
  Bus Creator/1 -> ACdat/1
  THB_COLD_IN/1 -> cooling/2(THB_COLD_IN), Bus Selector2/1
  THB_GEN_IN/1 -> Bus Selector/1, generator/1(THB_GEN_IN)
  generator/1(THV_GEN_OUT) -> THB_GEN_OUT/1
  THB_RC_IN/1 -> Bus Selector1/1, Bus Selector3/1, recooling/2(THB_RC_IN)
  Bus Selector1/1 -> Lookup_table Q_hot + Q_cold + Recooling/2(T_RC_IN)  "<Temperature>"
  recooling/1(THB_RC_OUT) -> THB_RC_OUT/1
  cooling/1(THB_COLD_OUT) -> THB_COLD_OUT/1
  Ctrl/1 -> Lookup_table Q_hot + Q_cold + Recooling/4(control), Bus Creator/4, Gain/1  "ControlSetpoint"
  Bus Selector2/1 -> Lookup_table Q_hot + Q_cold + Recooling/3(T_COLD_IN)  "<Temperature>"
  Lookup_table Q_hot + Q_cold + Recooling/2(Q_cold_kW) -> cooling/1(Q_cold), Bus Creator/1  "QdotCold"
  Lookup_table Q_hot + Q_cold + Recooling/1(Q_hot_kW) -> generator/2(Q_hot)
  Lookup_table Q_hot + Q_cold + Recooling/3(Q_recooling_kW) -> recooling/1(Q_recooling)
  el. consumption solutionpump [W]/1 -> Bus Creator/3  "Pel"
  CompareToZero/1 -> el. consumption solutionpump [W]/1
  Bus Selector/1 -> Lookup_table Q_hot + Q_cold + Recooling/1(T_GEN_IN)  "<Temperature>"
  Lookup_table Q_hot + Q_cold + Recooling/4(COP) -> Bus Creator/2  "COP"
  Bus Selector3/1 -> CompareToZero/1  "<MassFlow>"

== system carnot/Source/Chiller/Absorption_Chiller_ddT ==
  note: G = generator
      | E = evaporator
      | A = absorber
      | C = condenser
  THBload_in : Inport
  THBhot_in : Inport  Port=2
  THBcool_in : Inport  Port=3
  Ctrl : Inport  Port=4
  Bus Selector : BusSelector  OutputSignals=Temperature
  Bus Selector1 : BusSelector  OutputSignals=Temperature
  Mux : Mux  Inputs=2
  Pel_pump : Gain  Gain=Pel_p
  Tcool_in_max : Relay  OnSwitchValue=35  OffSwitchValue=30  OnOutputValue=0  OffOutputValue=1
  Tload_out_min : Relay  OnSwitchValue=2  OffSwitchValue=0
  Transfer Fcn (with initial states) : Subsystem  mask(Transfer Function with Initial States){N=[1], D=[10 1], X0=20}
      mask prompts: N "Numerator:"; D "Denominator:"; X0 "Initial conditions:"
      mask help: Vector expressions for numerator, and denominator. Coefficients are in descending powers of s.
      mask init:
      | [A,B,C,Dd]=tf2ss(N,D);if (isempty(X0));[m,n]=size(A);X0=zeros(1,m); end;
      mask Help: Specify the initial states for the transfer function.  The state ordering is determined by the m-file tf2ss.  There is no unique mapping of the states in a transfer function to states in a state-space representation.  However, tf2ss will consistently use the same mapping for a given transfer function.
      mask Display: dpoly(N,D,'s')
  absorber / condenser : Subsystem
  boiler : Subsystem
  deltadelta_t : Subsystem
  evaporator : Subsystem
  prod : Product  Inputs=3
  THBload : Outport
  THBhot_out : Outport  Port=2
  THBcool_out : Outport  Port=3
  Pel_Pump : Outport  Port=4
  Qdot : Outport  Port=5
  wires:
  Mux/1 -> Qdot/1
  Ctrl/1 -> prod/2, Pel_pump/1  "system on/off"
  Bus Selector/1 -> Tcool_in_max/1  "<Temperature>"
  Tcool_in_max/1 -> prod/3
  Transfer Fcn (with initial states)/1(Out1) -> Tload_out_min/1
  Bus Selector1/1 -> Transfer Fcn (with initial states)/1(In1)  "<Temperature>"
  prod/1 -> absorber / condenser/4(on), boiler/3(on), evaporator/3(on)
  Tload_out_min/1 -> prod/1
  Pel_pump/1 -> Pel_Pump/1
  absorber / condenser/2(t_AC) -> deltadelta_t/3(t_AC)
  boiler/2(t_B) -> deltadelta_t/1(t_B)
  evaporator/3(Qdot_E [W]) -> Mux/1, absorber / condenser/2(Qdot_E_act [W])
  evaporator/2(t_E) -> deltadelta_t/2(t_E)
  evaporator/1(THBload) -> Bus Selector1/1, THBload/1
  absorber / condenser/1(THBcooler) -> THBcool_out/1
  THBcool_in/1 -> Bus Selector/1, absorber / condenser/1(THBcooler_in)
  THBhot_in/1 -> boiler/1(THBhot_in)
  boiler/1(THVhot_out) -> THBhot_out/1
  THBload_in/1 -> evaporator/1(THBload_in)
  boiler/3(Qdot_G [W]) -> Mux/2, absorber / condenser/3(Qdot_G [W])
  deltadelta_t/1(deltadelta_t) -> boiler/2(deltadelta_t), evaporator/2(deltadelta_t)

== system carnot/Source/Chiller/Compression_Air_Water_Chiller ==
  THB_water_in : Inport
  T_AIR_IN : Inport  Port=2
  control : Inport  Port=3
  Lookup_tables _COP + Q_cold_faktor : Subsystem  TreatAsAtomicUnit=on
  cooling : Subsystem
  measure_T_WATER_OUT : Subsystem  mask(temperature measurement sensor){tc=10, t0=20}
      mask prompts: tc "time constant of sensor [s]"; t0 "initial temperature [degree centigrade]"
      mask help: Measurement sensor for temperatures with first-oder hold. Temperature is in degree centigrade.
      mask init:
      | tc = 1/max(tc, 0.001);
      mask Help: eval('htmlhelp (''chap_4_2m.htm#measure_T'')')
      mask Display: plot(-18,0,30,20,[0 20],[0 0],[10 10 8 8 12 12 10],[0 8 8 17 17 8 8],[10 10 9 9 11 11 10 9],[15 10 10 9 9 10 9 10])
  THB_water_out : Outport
  COP : Outport  Port=2
  P_el : Outport  Port=3
  Q_cold : Outport  Port=4
  wires:
  THB_water_in/1 -> cooling/1(THB_in)
  Lookup_tables _COP + Q_cold_faktor/2(Q_cold) -> cooling/2(Q_cold), Q_cold/1
  T_AIR_IN/1 -> Lookup_tables _COP + Q_cold_faktor/1(T_AIR_IN)
  cooling/1(THB_out) -> measure_T_WATER_OUT/1(THV_in)
  measure_T_WATER_OUT/2(THV) -> THB_water_out/1
  measure_T_WATER_OUT/1(T) -> Lookup_tables _COP + Q_cold_faktor/2(T_WATER_OUT)
  control/1 -> Lookup_tables _COP + Q_cold_faktor/3(control_AC)
  Lookup_tables _COP + Q_cold_faktor/3(P_el) -> P_el/1
  Lookup_tables _COP + Q_cold_faktor/1(COP) -> COP/1

== system carnot/Source/Chiller/Cooling_Tower ==
  note: Kaltwassertemperatur bei
      | 100% Luftdurchsatz
      | 30% Glykolgehalt
      | 2,4 l/s Prozessfluid-Volumenstrom
  note: --Indizes--
      | FK - Feuchtkugel
      | l - Luft
      | i - Prozessfluid
      | e - ein
      | a - aus
      |
      |
      | --Abkürzungen--
      | cp - spezifische Wärmekapazität
      | n/rpm - Drehzahl
      | p - Druck
      | P - Leistung
      | t - Temperatur
      | phi - relative Feuchte
      | x - absolute Feuchte
      | control - Steuersignal
      | mdot - Massenstrom
      | Qdot - Rückkühlleistung
      | vdot - Volumenstrom
  THBin : Inport
  WDB : Inport  Port=2
  rpm_fan : Inport  Port=3
  control_fan : Inport  Port=4
  Bus Creator : BusCreator  Inputs=10
  Bus Selector : BusSelector  OutputSignals=Temperature_Ambient,Relative_Humidity
  Bus Selector1 : BusSelector  OutputSignals=Tnodes
  Demux : Demux  Outputs=[1 1 1 1 1 1 14]
  Fan : Subsystem
  Feuchtkugel- temperatureinfluss / wet-bulb temperature effect : Subsystem
  Ground : Ground
  Heat_Capacity : $bdroot/Basic/Material_Properties/Heat_Capacity  VariantControl=CarlibClassic  INPUTARGUMENTS=state variables (classic)  DEBUGLEVEL=DEBUGLEVEL  MAXTOTALWARNINGS=inf  MAXCONSECUTIVEWARNINGS=inf  WRITETOFILE=0  FILENAME='errors.txt'
  Leistungseinflüsse / influence on coolingpower : Subsystem
  Mux : Mux  Inputs=7
  Storage_Type_0 : $bdroot/Storage/Thermal/Storage_Type_0  t0=20  hgt=0.95493  stgtype=0  mpts=[1 2 3 4 5]  tini=[20 20 20 20 20]  PathName=fullfile(path_carnot('libsl'),'Storage','Thermal','Storage_Type_0','parameter_set')  FileName='<user defined>'  userPath=off  userParam=on  uwall=1  ubot=1  utop=1  axcond=1  volume=0.03  dia=0.2  standing=standing cylinder  nodes=5  mpoints=5  Tsensor=0.5  pipe1inlet=1  pipe1outlet=0  pipe1dia=0.03  heater1start=0.2  heater1end=0.25
  THB2THV : $bdroot/Toolbox/THB2THV
  THV2THB : $bdroot/Toolbox/THV2THB
  Terminator1 : Terminator
  Verbrauch / consumption : Subsystem
  THBout : Outport
  data logging : Outport  Port=2
  wires:
  Ground/1 -> Storage_Type_0/3
  Bus Selector1/1 -> Bus Creator/10  "<Tnodes>"
  Storage_Type_0/1 -> Bus Selector1/1
  Storage_Type_0/2 -> Terminator1/1  "Tnodes"
  THB2THV/1 -> Demux/1
  THV2THB/1 -> Storage_Type_0/2
  Storage_Type_0/3 -> THBout/1
  THBin/1 -> THB2THV/1
  Demux/3 -> Leistungseinflüsse / influence on coolingpower/4(mdot_i), Mux/3  "mdot"
  Demux/7 -> Mux/7
  Demux/5 -> Heat_Capacity/3, Mux/5, Leistungseinflüsse / influence on coolingpower/5(Fluid_Type)  "fluid"
  Mux/1 -> THV2THB/1  "THV out"
  Demux/4 -> Heat_Capacity/2, Mux/4  "p"
  rpm_fan/1 -> Fan/1(n_fan), Bus Creator/4  "rpm fan [1/min]"
  Feuchtkugel- temperatureinfluss / wet-bulb temperature effect/3(dt) -> Heat_Capacity/1
  Feuchtkugel- temperatureinfluss / wet-bulb temperature effect/2(t_ia_FK) -> Leistungseinflüsse / influence on coolingpower/1(t_ia_FK)
  Demux/2 -> Feuchtkugel- temperatureinfluss / wet-bulb temperature effect/2(t_ie), Leistungseinflüsse / influence on coolingpower/3(t_ie), Verbrauch / consumption/7(t_ie)  "T"
  Leistungseinflüsse / influence on coolingpower/2(t_ia_ist) -> Mux/2
  Heat_Capacity/1 -> Leistungseinflüsse / influence on coolingpower/2(cp_i)
  Fan/2(vdot_fan) -> Verbrauch / consumption/2(vdot_fan), Bus Creator/3  "v_dot_fan"
  Verbrauch / consumption/2(power) -> Bus Creator/8  "power ct"
  Fan/3(P_fan) -> Verbrauch / consumption/3(P_fan)
  control_fan/1 -> Verbrauch / consumption/4(control_fan), Leistungseinflüsse / influence on coolingpower/Enable, Feuchtkugel- temperatureinfluss / wet-bulb temperature effect/Enable
  Demux/1 -> Mux/1  "ID"
  Feuchtkugel- temperatureinfluss / wet-bulb temperature effect/1(t_FK) -> Bus Creator/1  "wet-bulb temperature"
  Leistungseinflüsse / influence on coolingpower/1(Qdot_i_ist) -> Verbrauch / consumption/1(Qdot)  "Q_i_ist"
  Fan/1(n_fan [%]) -> Leistungseinflüsse / influence on coolingpower/7(n_fan [%]), Bus Creator/2  "rpm fan [%]"
  Bus Selector/2 -> Verbrauch / consumption/5(phi_le), Bus Creator/5  "<Relative_Humidity>"
  Bus Selector/1 -> Verbrauch / consumption/6(t_le), Bus Creator/6, Storage_Type_0/1  "<Temperature_Ambient>"
  Verbrauch / consumption/3(Wasserverbrauch) -> Bus Creator/9  "water consumption"
  Demux/6 -> Heat_Capacity/4, Leistungseinflüsse / influence on coolingpower/6(Fluid_mix), Mux/6  "mix"
  WDB/1 -> Feuchtkugel- temperatureinfluss / wet-bulb temperature effect/1(WDB), Bus Selector/1
  Bus Creator/1 -> data logging/1
  Verbrauch / consumption/1(energy) -> Bus Creator/7  "energy ct"

== system carnot/Source/Cogeneration/microCHP_constant ==
  THBreturn : Inport
  control : Inport  Port=2
  Bus Creator : BusCreator  Inputs=8
  Demux : Demux  Outputs=[1 1 1 1 1 1]
  Demux3 : Demux  Outputs=[6 14]
  Divide2 : Product  Inputs=*/
  Dot Prodct1 : DotProduct  InputSameDT=on  OutDataTypeStr=Inherit: Inherit via internal rule
  Dot Prodct2 : DotProduct  InputSameDT=on  OutDataTypeStr=Inherit: Inherit via internal rule
  Dot Product1 : DotProduct  InputSameDT=on  OutDataTypeStr=Inherit: Inherit via internal rule
  Ground : Ground
  Heat_Capacity : $bdroot/Basic/Material_Properties/Heat_Capacity  VariantControl=CarlibClassic  INPUTARGUMENTS=state variables (classic)  DEBUGLEVEL=DEBUGLEVEL  MAXTOTALWARNINGS=inf  MAXCONSECUTIVEWARNINGS=inf  WRITETOFILE=0  FILENAME='errors.txt'
  MinMax : MinMax  Inputs=2
  Mux1 : Mux  Inputs=[1 1 1 1 1 1 14]
  P_el : Constant  Value=P_el
  P_fuel : Constant  Value=P_fuel
  P_th : Constant  Value=P_th
  P_th_base : Constant  Value=11520
  P_th_factor-lookup-table : Lookup_n-D  NumberOfTableDimensions=1  BreakpointsForDimension1=[45,50,60,65,74]  BreakpointsForDimension2=[44,80]  BreakpointsForDimension3=[1:2]  BreakpointsForDimension4=[1:2]  Table=[1.09 1.06 1 0.98 0.94]  InputSameDT=on
  Product : Product  Inputs=//**  SaturateOnIntegerOverflow=on  RndMeth=Zero  InputSameDT=on  OutDataTypeStr=Inherit: Same as first input
  Relay : Relay  OnSwitchValue=T_return_max  OffSwitchValue=T_return_max-1  OnOutputValue=0  OffOutputValue=1
  Storage_Type_0 : $bdroot/Storage/Thermal/Storage_Type_0  t0=25  hgt=0.63662  stgtype=0  mpts=[1 2 3 4 5 6 7 8 9 10]  tini=[25 25 25 25 25 25 25 25 25 25]  PathName=fullfile(path_carnot('libsl'),'Storage','Thermal','Storage_Type_0','parameter_set')  FileName='<user defined>'  userPath=off  userParam=on  uwall=1  ubot=1  utop=1  axcond=1  volume=0.02  dia=0.2  standing=standing cylinder  nodes=10  mpoints=10  Tsensor=0.5  pipe1inlet=1  pipe1outlet=0  pipe1dia=0.03  heater1start=0.2  heater1end=0.25
  Sum : Sum  SaturateOnIntegerOverflow=on  InputSameDT=on  OutDataTypeStr=Inherit: Same as first input
  THB2THV : $bdroot/Toolbox/THB2THV
  THV2THB : $bdroot/Toolbox/THV2THB
  T_amb : Constant  Value=15
  Terminator : Terminator
  Terminator1 : Terminator
  energy and efficiency : Subsystem
  measure_T : Subsystem  mask(temperature measurement sensor){tc=10, t0=25}
      mask prompts: tc "time constant of sensor [s]"; t0 "initial temperature [degree centigrade]"
      mask help: Measurement sensor for temperatures with first-oder hold. Temperature is in degree centigrade.
      mask init:
      | tc = 1/max(tc, 0.001);
      mask Help: eval('man (''measure_T'')')
      mask Display: plot(-18,0,30,20,[0 20],[0 0],[10 10 8 8 12 12 10],[0 8 8 17 17 8 8],[10 10 9 9 11 11 10 9],[15 10 10 9 9 10 9 10])
  pump and return temperature raising facility : Subsystem  mask(Pump and return temperature raising facility){fluid_id=water, mix=0, dia=0.02, power=100, p0=3e5}
      mask prompts: fluid_id "fluid"; mix "percentage of fluid mix [0..1]"; dia "diameter at in- and outlet [m]"; power "electric power consumption [W]"; p0 "system pressure [Pa]"
      mask help:
      | In this modul a pump and a return temperature raising facility are modelled by two lookup-tables. They are based on measured data.
      |
      | The mass flow-lookup table gives out the mass flow (outside of CHP) depending on the return flow temperature T_return (outside of CHP). The return flow temperature (inside of CHP) is kept on 74°C by means of a thermostatic mixing valve.
      |
      | The T_flow-lookup table gives out the flow temperature T_flow depending on the return flow temperature (outside of CHP).
      |
      | The mass flow (outside of CHP) varies by means of multiplication with a factor f_flowSetpoint depending on the flow setpoint temperature T_flowSetpoint.
      | f_flowSetpoint is calculated according to the following formula:
      | (T_flow-T_return)/(T_flowSetpoint-T_return).
      |
      | The mass flow (outside of CHP) depends also on the nominal heating power P_heating and is therefor multiplied with a factor f_power.
      | f_power is calculated according to the following formula: P_heating/11520.
      mask init:
      | mix = min(1, max(0, mix));
      | dia = max(0.001, dia);
      | p0 = max(p0, 1e5);
      mask Help: eval('htmlhelp (''chap_4_2p.htm#pump_const'')')
      mask TypeOptions fluid_id: water | air | cotton_oil | silicone_oil | water_glycol_mix
      mask Display: plot(0,0,100,100,[40,70,40,30,30,40,60,70,70,60,40],[70,50,30,40,60,70,70,60,40,30,30])
  zeroavoiding : Saturate  UpperLimit=inf  LowerLimit=1e-5
  THBflow : Outport
  data : Outport  Port=2
  wires:
  Ground/1 -> Storage_Type_0/3
  Storage_Type_0/2 -> Terminator1/1
  Relay/1 -> MinMax/1
  Bus Creator/1 -> data/1
  measure_T/1(THV) -> pump and return temperature raising facility/1(THVin)
  Dot Prodct2/1 -> energy and efficiency/3(P_gas)
  Divide2/1 -> Dot Prodct2/1, Dot Prodct1/1
  P_el/1 -> Dot Prodct1/2
  Dot Prodct1/1 -> energy and efficiency/4(P_el)
  P_fuel/1 -> Dot Prodct2/2
  P_th_base/1 -> Divide2/2
  MinMax/1 -> Bus Creator/7, energy and efficiency/2(control_CHP), Product/4, pump and return temperature raising facility/2(control)  "ControlActual"
  Dot Product1/1 -> energy and efficiency/1(P_th), Product/3
  measure_T/2(T) -> Relay/1
  Demux/2 -> Sum/1, Heat_Capacity/1, P_th_factor-lookup-table/1  "T"
  Product/1 -> Sum/2
  pump and return temperature raising facility/1(THV) -> Demux3/1
  THBreturn/1 -> THB2THV/1
  P_th/1 -> Divide2/1, Dot Product1/2
  P_th_factor-lookup-table/1 -> Dot Product1/1
  Mux1/1 -> THV2THB/1
  Demux3/2 -> Mux1/7
  Demux3/1 -> Demux/1
  Sum/1 -> Mux1/2
  zeroavoiding/1 -> Product/1
  Demux/3 -> zeroavoiding/1, Mux1/3  "mdot"
  Heat_Capacity/1 -> Product/2
  Demux/6 -> Mux1/6, Heat_Capacity/4
  Demux/5 -> Mux1/5, Heat_Capacity/3
  Demux/1 -> Mux1/1  "ID"
  Demux/4 -> Mux1/4, Heat_Capacity/2  "p"
  THV2THB/1 -> Storage_Type_0/2
  THB2THV/1 -> measure_T/1(THV_in)
  Storage_Type_0/3 -> THBflow/1
  Storage_Type_0/1 -> Terminator/1
  T_amb/1 -> Storage_Type_0/1
  energy and efficiency/6(eta_sys) -> Bus Creator/6  "eta_sys"
  energy and efficiency/5(eta_el) -> Bus Creator/5  "eta_el"
  energy and efficiency/4(eta_th) -> Bus Creator/4  "eta_th"
  energy and efficiency/3(Q_Gas) -> Bus Creator/3  "Q_Gas"
  energy and efficiency/2(Q_el) -> Bus Creator/2  "Q_el"
  energy and efficiency/1(Q_th) -> Bus Creator/1  "Q_th"
  control/1 -> Bus Creator/8, MinMax/2  "ControlSetpoint"
